simulink model "CoEng_Mon"  (R2016b)
settings: configuration reference "CodeGenConfigSet" (kept outside this file)
libraries: simulink x14
settings Model: Creator=lenovo  LastModifiedBy=Administrator
settings ConfigSetRef: SourceLocation=Base Workspace

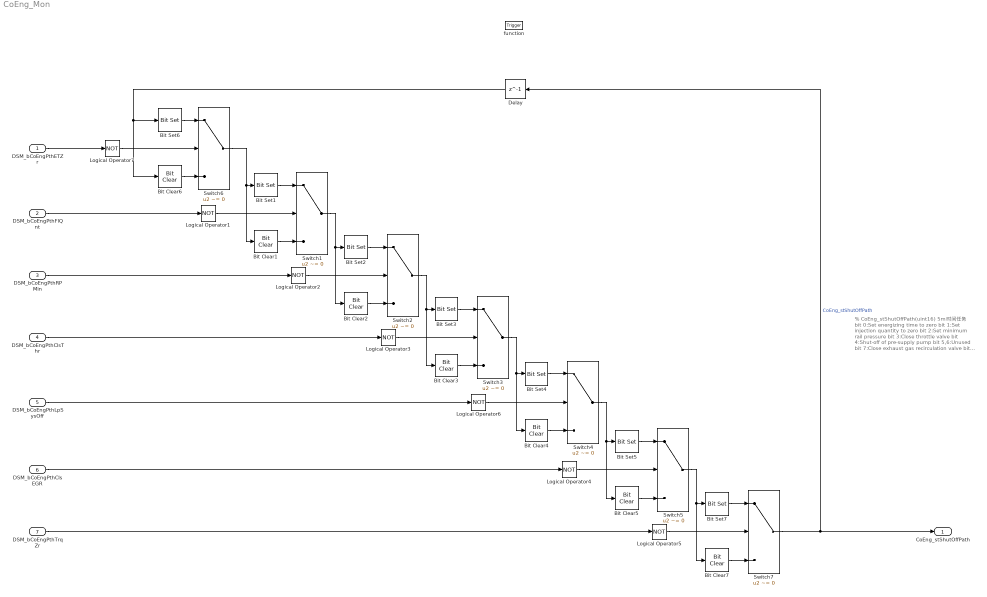
== system CoEng_Mon ==
  note: % CoEng_stShutOffPath(uint16) 5ms时间任务
      | bit 0:Set energizing time to zero
      | bit 1:Set injection quantity to zero
      | bit 2:Set minimum rail pressure
      | bit 3:Close throttle valve
      | bit 4:Shut-off of pre-supply pump
      | bit 5,6:Unused
      | bit 7:Close exhaust gas recirculation valve
      | bit 8:Set inner torque to zero %
  DSM_bCoEngPthETZr : Inport  Description=state of FId_CoEngPthETZr  OutMin=0  OutMax=1  OutDataTypeStr=boolean
  DSM_bCoEngPthFlQnt : Inport  Description=state of FId_CoEngPthFlQnt  Port=2  OutMin=0  OutMax=1  OutDataTypeStr=boolean
  DSM_bCoEngPthRPMin : Inport  Description=state of FId_CoEngPthRPMin  Port=3  OutMin=0  OutMax=1  OutDataTypeStr=boolean
  DSM_bCoEngPthClsThr : Inport  Description=state of FId_CoEngPthClsThr  Port=4  OutMin=0  OutMax=1  OutDataTypeStr=boolean
  DSM_bCoEngPthLpSysOff : Inport  Description=state of FId_CoEngPthLpSysOff  Port=5  OutMin=0  OutMax=1  OutDataTypeStr=boolean
  DSM_bCoEngPthClsEGR : Inport  Description=state of FId_CoEngPthClsEGR  Port=6  OutMin=0  OutMax=1  OutDataTypeStr=boolean
  DSM_bCoEngPthTrqZr : Inport  Description=state of FId_CoEngPthTrqZr  Port=7  OutMin=0  OutMax=1  OutDataTypeStr=boolean
  function : TriggerPort  TriggerType=function-call  VariantControl=Variant
  Bit Clear1 : simulink/Logic and Bit Operations/Bit Clear  iBit=1
  Bit Clear2 : simulink/Logic and Bit Operations/Bit Clear  iBit=2
  Bit Clear3 : simulink/Logic and Bit Operations/Bit Clear  iBit=3
  Bit Clear4 : simulink/Logic and Bit Operations/Bit Clear  iBit=4
  Bit Clear5 : simulink/Logic and Bit Operations/Bit Clear  iBit=7
  Bit Clear6 : simulink/Logic and Bit Operations/Bit Clear  iBit=0
  Bit Clear7 : simulink/Logic and Bit Operations/Bit Clear  iBit=8
  Bit Set1 : simulink/Logic and Bit Operations/Bit Set  iBit=1
  Bit Set2 : simulink/Logic and Bit Operations/Bit Set  iBit=2
  Bit Set3 : simulink/Logic and Bit Operations/Bit Set  iBit=3
  Bit Set4 : simulink/Logic and Bit Operations/Bit Set  iBit=4
  Bit Set5 : simulink/Logic and Bit Operations/Bit Set  iBit=7
  Bit Set6 : simulink/Logic and Bit Operations/Bit Set  iBit=0
  Bit Set7 : simulink/Logic and Bit Operations/Bit Set  iBit=8
  Delay : Delay  DelayLength=1  InitialCondition=0
  Logical Operator{1..7} (7 alike) : Logic  Operator=NOT  OutDataTypeStr=boolean
  Switch{1..7} (7 alike) : Switch  Criteria=u2 ~= 0
  CoEng_stShutOffPath : Outport  Description=Active shut-off paths resulting from active reversible,irreversible and afterrun shut-off paths  OutMin=0  OutMax=65535  OutDataTypeStr=State_uint16
  wires:
  Delay/1 -> Bit Set6/1, Bit Clear6/1
  Switch7/1 -> CoEng_stShutOffPath/1, Delay/1  "CoEng_stShutOffPath"
  Switch3/1 -> Bit Set4/1, Bit Clear4/1
  DSM_bCoEngPthTrqZr/1 -> Logical Operator5/1
  Bit Set7/1 -> Switch7/1
  Logical Operator5/1 -> Switch7/2
  Bit Clear7/1 -> Switch7/3
  Switch5/1 -> Bit Set7/1, Bit Clear7/1
  Bit Set5/1 -> Switch5/1
  DSM_bCoEngPthClsEGR/1 -> Logical Operator4/1
  Logical Operator4/1 -> Switch5/2
  Bit Clear5/1 -> Switch5/3
  Switch4/1 -> Bit Set5/1, Bit Clear5/1
  Bit Set4/1 -> Switch4/1
  Bit Clear4/1 -> Switch4/3
  DSM_bCoEngPthClsThr/1 -> Logical Operator3/1
  Bit Set3/1 -> Switch3/1
  Logical Operator3/1 -> Switch3/2
  Bit Clear3/1 -> Switch3/3
  Switch2/1 -> Bit Clear3/1, Bit Set3/1
  Bit Set2/1 -> Switch2/1
  DSM_bCoEngPthRPMin/1 -> Logical Operator2/1
  Logical Operator2/1 -> Switch2/2
  Bit Clear2/1 -> Switch2/3
  Switch1/1 -> Bit Clear2/1, Bit Set2/1
  DSM_bCoEngPthFlQnt/1 -> Logical Operator1/1
  Logical Operator1/1 -> Switch1/2
  Bit Set1/1 -> Switch1/1
  Bit Clear1/1 -> Switch1/3
  Logical Operator7/1 -> Switch6/2
  DSM_bCoEngPthETZr/1 -> Logical Operator7/1
  Bit Set6/1 -> Switch6/1
  Bit Clear6/1 -> Switch6/3
  Switch6/1 -> Bit Set1/1, Bit Clear1/1
  DSM_bCoEngPthLpSysOff/1 -> Logical Operator6/1
  Logical Operator6/1 -> Switch4/2
